simulink model "transfer_function_problem6"  (R2022a)
settings: Solver=VariableStepAuto  StartTime=0.0  StopTime=10.0  RelTol=1e-3
settings Model: Creator=prafu  LastModifiedBy=prafu

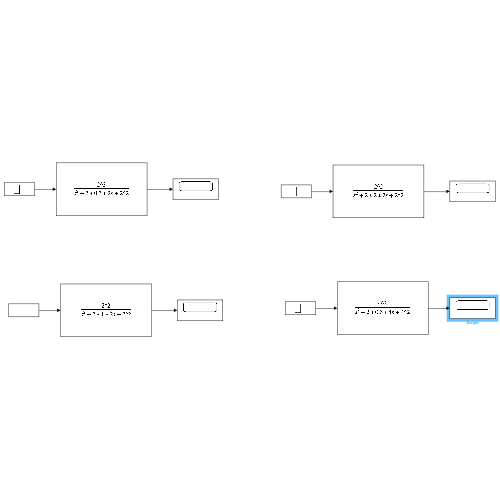
[thumbnail: Simulink's stored preview of the top-level diagram]
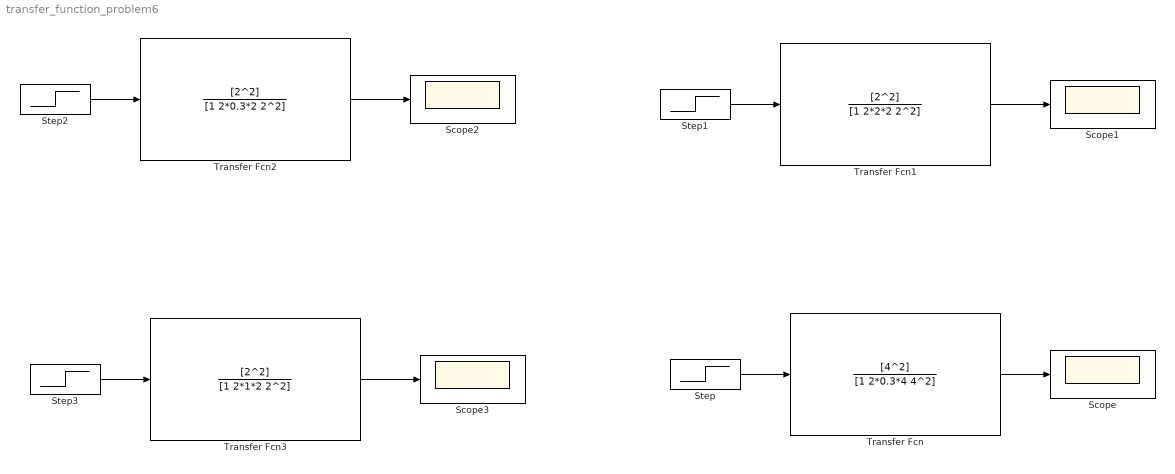
== system transfer_function_problem6 ==
  Scope{,1..3} (4 alike) : Scope
  Step{,1..3} (4 alike) : Step  SampleTime=0
  Transfer Fcn : TransferFcn  Numerator=[4^2]  Denominator=[1 2*0.3*4 4^2]
  Transfer Fcn1 : TransferFcn  Numerator=[2^2]  Denominator=[1 2*2*2 2^2]
  Transfer Fcn2 : TransferFcn  Numerator=[2^2]  Denominator=[1 2*0.3*2 2^2]
  Transfer Fcn3 : TransferFcn  Numerator=[2^2]  Denominator=[1 2*1*2 2^2]
  wires:
  Step/1 -> Transfer Fcn/1
  Transfer Fcn/1 -> Scope/1
  Step1/1 -> Transfer Fcn1/1
  Transfer Fcn1/1 -> Scope1/1
  Transfer Fcn2/1 -> Scope2/1
  Step2/1 -> Transfer Fcn2/1
  Step3/1 -> Transfer Fcn3/1
  Transfer Fcn3/1 -> Scope3/1
